simulink model "Model_V5"  (R2024b)
settings: Solver=VariableStepAuto  StartTime=0.0  StopTime=3600*12  RelTol=1e-3
undefined symbols (not defined in the file): PropsSI
libraries: fl_lib x569, SimscapeFluids_lib x61, nesl_utility x27
(part 4 of 7)

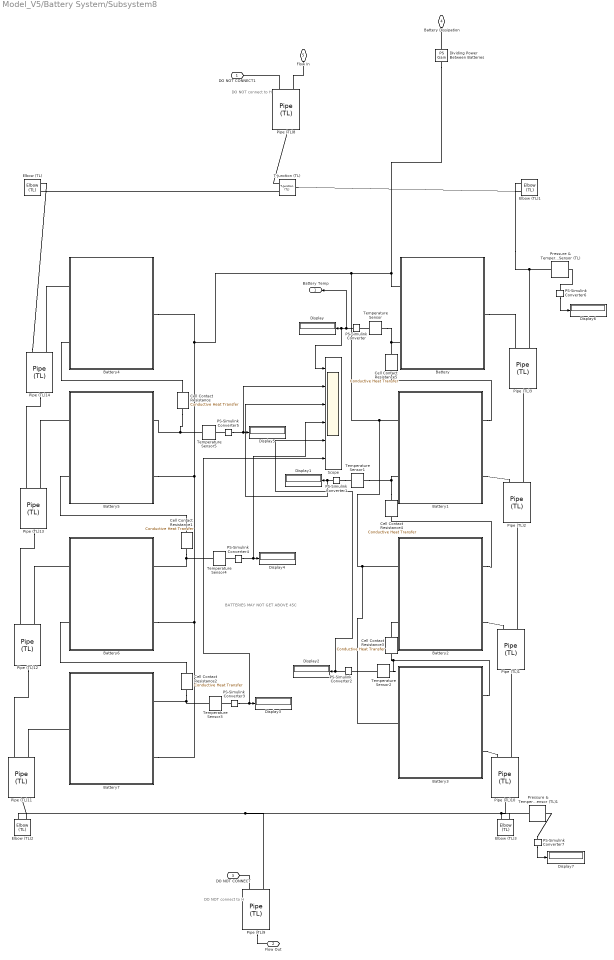
== system Model_V5/Battery System/Subsystem8 ==
  note: BATTERIES MAY NOT GET ABOVE 45C
  note: DO NOT connect to H
  note: DO NOT connect to H
  Battery : Subsystem
      settings: PortSchema="{\"entries\":[{\"content\":{\"sides\":[{\"content\":{},\"type\":\"ConnectorPlacement.EquallySpacedRectSide\",\"uuid\":\"c3611117-ee8e-4b0c-a918-53f59eb75c39\"},{\"content\":{\"side\":\"RIGHT\"},\"type\":\"ConnectorPlacement.EquallySpacedRectSide\",\"uuid\":\"d30ab4df-cb16-40c1-971c-28ba623de8c6\"},{\"content\":{\"connectorIds\":[\"LConn1\",\"LConn2\"],\"side\":\"TOP\"},\"type\":\"ConnectorPlacement.EquallySpacedRectSide\",\"uuid\":\"583a14bc-e521-4cb2-80b3-70b113bba0cc\"},{\"content\":{\"connectorIds\":[\"RConn1\"],\"side\":\"BOTTOM\"},\"type\":\"ConnectorPlacement.EquallySpacedRectSide\",\"uuid\":\"e76e2aad-c8ca-4e56-91e9-6eb1fa374ff6\"}]},\"type\":\"ConnectorPlacement.EquallySpacedConnector\",\"uuid\":\"b27f219d-6435-4727-95fa-791c0451b06d\"}],\"packageUris\":[\"http://schema.mathworks.com/mf0/Connector/R2020b\"],\"version\":\"1.0\"}"
  Battery1 : Subsystem
      settings: PortSchema="{\"entries\":[{\"content\":{\"sides\":[{\"content\":{},\"type\":\"ConnectorPlacement.EquallySpacedRectSide\",\"uuid\":\"c3611117-ee8e-4b0c-a918-53f59eb75c39\"},{\"content\":{\"side\":\"RIGHT\"},\"type\":\"ConnectorPlacement.EquallySpacedRectSide\",\"uuid\":\"d30ab4df-cb16-40c1-971c-28ba623de8c6\"},{\"content\":{\"connectorIds\":[\"LConn1\",\"LConn2\"],\"side\":\"TOP\"},\"type\":\"ConnectorPlacement.EquallySpacedRectSide\",\"uuid\":\"583a14bc-e521-4cb2-80b3-70b113bba0cc\"},{\"content\":{\"connectorIds\":[\"RConn1\",\"RConn2\"],\"side\":\"BOTTOM\"},\"type\":\"ConnectorPlacement.EquallySpacedRectSide\",\"uuid\":\"e76e2aad-c8ca-4e56-91e9-6eb1fa374ff6\"}]},\"type\":\"ConnectorPlacement.EquallySpacedConnector\",\"uuid\":\"b27f219d-6435-4727-95fa-791c0451b06d\"}],\"packageUris\":[\"http://schema.mathworks.com/mf0/Connector/R2020b\"],\"version\":\"1.0\"}"
  Battery2 : Subsystem
      settings: PortSchema="{\"entries\":[{\"content\":{\"sides\":[{\"content\":{},\"type\":\"ConnectorPlacement.EquallySpacedRectSide\",\"uuid\":\"c3611117-ee8e-4b0c-a918-53f59eb75c39\"},{\"content\":{\"side\":\"RIGHT\"},\"type\":\"ConnectorPlacement.EquallySpacedRectSide\",\"uuid\":\"d30ab4df-cb16-40c1-971c-28ba623de8c6\"},{\"content\":{\"connectorIds\":[\"LConn1\",\"LConn2\"],\"side\":\"TOP\"},\"type\":\"ConnectorPlacement.EquallySpacedRectSide\",\"uuid\":\"583a14bc-e521-4cb2-80b3-70b113bba0cc\"},{\"content\":{\"connectorIds\":[\"RConn1\",\"RConn2\"],\"side\":\"BOTTOM\"},\"type\":\"ConnectorPlacement.EquallySpacedRectSide\",\"uuid\":\"e76e2aad-c8ca-4e56-91e9-6eb1fa374ff6\"}]},\"type\":\"ConnectorPlacement.EquallySpacedConnector\",\"uuid\":\"b27f219d-6435-4727-95fa-791c0451b06d\"}],\"packageUris\":[\"http://schema.mathworks.com/mf0/Connector/R2020b\"],\"version\":\"1.0\"}"
  Battery3 : Subsystem
      settings: PortSchema="{\"entries\":[{\"content\":{\"sides\":[{\"content\":{},\"type\":\"ConnectorPlacement.EquallySpacedRectSide\",\"uuid\":\"c3611117-ee8e-4b0c-a918-53f59eb75c39\"},{\"content\":{\"side\":\"RIGHT\"},\"type\":\"ConnectorPlacement.EquallySpacedRectSide\",\"uuid\":\"d30ab4df-cb16-40c1-971c-28ba623de8c6\"},{\"content\":{\"connectorIds\":[\"LConn1\"],\"side\":\"TOP\"},\"type\":\"ConnectorPlacement.EquallySpacedRectSide\",\"uuid\":\"583a14bc-e521-4cb2-80b3-70b113bba0cc\"},{\"content\":{\"connectorIds\":[\"RConn1\",\"RConn2\"],\"side\":\"BOTTOM\"},\"type\":\"ConnectorPlacement.EquallySpacedRectSide\",\"uuid\":\"e76e2aad-c8ca-4e56-91e9-6eb1fa374ff6\"}]},\"type\":\"ConnectorPlacement.EquallySpacedConnector\",\"uuid\":\"b27f219d-6435-4727-95fa-791c0451b06d\"}],\"packageUris\":[\"http://schema.mathworks.com/mf0/Connector/R2020b\"],\"version\":\"1.0\"}"
  Battery4 : Subsystem
      settings: PortSchema="{\"entries\":[{\"content\":{\"sides\":[{\"content\":{},\"type\":\"ConnectorPlacement.EquallySpacedRectSide\",\"uuid\":\"c3611117-ee8e-4b0c-a918-53f59eb75c39\"},{\"content\":{\"side\":\"RIGHT\"},\"type\":\"ConnectorPlacement.EquallySpacedRectSide\",\"uuid\":\"d30ab4df-cb16-40c1-971c-28ba623de8c6\"},{\"content\":{\"connectorIds\":[\"LConn1\"],\"side\":\"TOP\"},\"type\":\"ConnectorPlacement.EquallySpacedRectSide\",\"uuid\":\"583a14bc-e521-4cb2-80b3-70b113bba0cc\"},{\"content\":{\"connectorIds\":[\"RConn1\",\"RConn2\"],\"side\":\"BOTTOM\"},\"type\":\"ConnectorPlacement.EquallySpacedRectSide\",\"uuid\":\"e76e2aad-c8ca-4e56-91e9-6eb1fa374ff6\"}]},\"type\":\"ConnectorPlacement.EquallySpacedConnector\",\"uuid\":\"b27f219d-6435-4727-95fa-791c0451b06d\"}],\"packageUris\":[\"http://schema.mathworks.com/mf0/Connector/R2020b\"],\"version\":\"1.0\"}"
  Battery5 : Subsystem
      settings: PortSchema="{\"entries\":[{\"content\":{\"sides\":[{\"content\":{},\"type\":\"ConnectorPlacement.EquallySpacedRectSide\",\"uuid\":\"c3611117-ee8e-4b0c-a918-53f59eb75c39\"},{\"content\":{\"side\":\"RIGHT\"},\"type\":\"ConnectorPlacement.EquallySpacedRectSide\",\"uuid\":\"d30ab4df-cb16-40c1-971c-28ba623de8c6\"},{\"content\":{\"connectorIds\":[\"LConn1\",\"LConn2\"],\"side\":\"TOP\"},\"type\":\"ConnectorPlacement.EquallySpacedRectSide\",\"uuid\":\"583a14bc-e521-4cb2-80b3-70b113bba0cc\"},{\"content\":{\"connectorIds\":[\"RConn1\",\"RConn2\"],\"side\":\"BOTTOM\"},\"type\":\"ConnectorPlacement.EquallySpacedRectSide\",\"uuid\":\"e76e2aad-c8ca-4e56-91e9-6eb1fa374ff6\"}]},\"type\":\"ConnectorPlacement.EquallySpacedConnector\",\"uuid\":\"b27f219d-6435-4727-95fa-791c0451b06d\"}],\"packageUris\":[\"http://schema.mathworks.com/mf0/Connector/R2020b\"],\"version\":\"1.0\"}"
  Battery6 : Subsystem
      settings: PortSchema="{\"entries\":[{\"content\":{\"sides\":[{\"content\":{},\"type\":\"ConnectorPlacement.EquallySpacedRectSide\",\"uuid\":\"c3611117-ee8e-4b0c-a918-53f59eb75c39\"},{\"content\":{\"side\":\"RIGHT\"},\"type\":\"ConnectorPlacement.EquallySpacedRectSide\",\"uuid\":\"d30ab4df-cb16-40c1-971c-28ba623de8c6\"},{\"content\":{\"connectorIds\":[\"LConn1\",\"LConn2\"],\"side\":\"TOP\"},\"type\":\"ConnectorPlacement.EquallySpacedRectSide\",\"uuid\":\"583a14bc-e521-4cb2-80b3-70b113bba0cc\"},{\"content\":{\"connectorIds\":[\"RConn1\",\"RConn2\"],\"side\":\"BOTTOM\"},\"type\":\"ConnectorPlacement.EquallySpacedRectSide\",\"uuid\":\"e76e2aad-c8ca-4e56-91e9-6eb1fa374ff6\"}]},\"type\":\"ConnectorPlacement.EquallySpacedConnector\",\"uuid\":\"b27f219d-6435-4727-95fa-791c0451b06d\"}],\"packageUris\":[\"http://schema.mathworks.com/mf0/Connector/R2020b\"],\"version\":\"1.0\"}"
  Battery7 : Subsystem
      settings: PortSchema="{\"entries\":[{\"content\":{\"sides\":[{\"content\":{},\"type\":\"ConnectorPlacement.EquallySpacedRectSide\",\"uuid\":\"c3611117-ee8e-4b0c-a918-53f59eb75c39\"},{\"content\":{\"side\":\"RIGHT\"},\"type\":\"ConnectorPlacement.EquallySpacedRectSide\",\"uuid\":\"d30ab4df-cb16-40c1-971c-28ba623de8c6\"},{\"content\":{\"connectorIds\":[\"LConn1\",\"LConn2\"],\"side\":\"TOP\"},\"type\":\"ConnectorPlacement.EquallySpacedRectSide\",\"uuid\":\"583a14bc-e521-4cb2-80b3-70b113bba0cc\"},{\"content\":{\"connectorIds\":[\"RConn1\"],\"side\":\"BOTTOM\"},\"type\":\"ConnectorPlacement.EquallySpacedRectSide\",\"uuid\":\"e76e2aad-c8ca-4e56-91e9-6eb1fa374ff6\"}]},\"type\":\"ConnectorPlacement.EquallySpacedConnector\",\"uuid\":\"b27f219d-6435-4727-95fa-791c0451b06d\"}],\"packageUris\":[\"http://schema.mathworks.com/mf0/Connector/R2020b\"],\"version\":\"1.0\"}"
  Cell Contact Resistance{,1..5} (6 alike) : fl_lib/Thermal/Thermal Elements/Conductive Heat Transfer  thermal_type=foundation.enum.ConstantVariableTabulated.Constant  wall_geometry=foundation.enum.ConductionWallGeometry.Planar  area=12*12 mm^2  thickness=0.003 in  d_in=0.05 m  d_out=0.1 m  L=1 m  th_cond_min=10 W/(K*m)  th_cond=1.38 W/(K*m)  th_cond_TLU=[413, 401, 392, 383, 371, 357, 342] W/(K*m)  temp_TLU=[200, 273, 400, 600, 800, 1000, 1200] K  T_specify=off  T_priority=None  T=0 K  T_nominal_specify=off  T_nominal_value=1  T_nominal_unit=K  Q_specify=off  Q_priority=None  Q=0 W  Q_nominal_specify=off  Q_nominal_value=1  Q_nominal_unit=W
  Display{,1..7} (8 alike) : Display
  Dividing Power Between Batteries : fl_lib/Physical Signals/Functions/PS Gain  gain=1/8
  Elbow (TL){,1..3} (4 alike) : SimscapeFluids_lib/Thermal Liquid/Pipes & Fittings/Elbow (TL)  elbow_type=fluids.thermal_liquid.pipes_fittings.enum.ElbowType.Smooth  diameter_elbow=1.5 in  angle_elbow=90 deg  Re_c=150
      settings: InternalSimscapePortConfiguration="{\"Bottom\":[],\"Left\":[{\"id\":\"A\",\"label\":\"A\",\"type\":\"foundation.thermal_liquid.thermal_liquid\"}],\"Right\":[],\"Top\":[{\"id\":\"B\",\"label\":\"B\",\"type\":\"foundation.thermal_liquid.thermal_liquid\"}]}"
  PS-Simulink Converter{,1..7} (8 alike) : nesl_utility/PS-Simulink Converter  PhysicalDomain=network_engine_domain  SubClassName=ps_output  LeftPortType=input  RightPortType=output  PseudoPeriodic=off  Frequencies=[]  VectorFormat=inherit  Unit=degC  AffineConversion=on
  Pipe (TL)1 : fl_lib/Thermal Liquid/Elements/Pipe (TL)  length=5*301.576 mm  area=5*(99.7+500)*(500+11.6) mm^2  Dh=(10*(99.7+500)*(500+11.6))/((5*(11.6+500))+(99.7+500)) mm  length_add=1 m  roughness=15e-6 m  Re_lam=2000  Re_tur=4000  shape_factor=64  Nu_lam=3.66  dynamic_compressibility=true  inertia=false  p0=0.101325 MPa  T0=293.15 K  mdot0=0 kg/s
  Pipe (TL){10..14} (5 alike) : fl_lib/Thermal Liquid/Elements/Pipe (TL)  length=301.576*5 mm  area=5*(99.7+500)*(500+11.6) mm^2  Dh=(10*(99.7+500)*(500+11.6))/((5*(11.6+500))+(99.7+500)) mm  length_add=1 m  roughness=15e-6 m  Re_lam=2000  Re_tur=4000  shape_factor=64  Nu_lam=3.66  dynamic_compressibility=true  inertia=false  p0=0.101325 MPa  T0=293.15 K  mdot0=0 kg/s
  Pipe (TL)2 : fl_lib/Thermal Liquid/Elements/Pipe (TL)  length=5*301.576 mm  area=5*(99.7+500)*(500+11.6) mm^2  Dh=(10*(99.7+500)*(500+11.6))/((5*(11.6+500))+(99.7+500)) mm  length_add=1 m  roughness=15e-6 m  Re_lam=2000  Re_tur=4000  shape_factor=64  Nu_lam=3.66  dynamic_compressibility=true  inertia=false  p0=0.101325 MPa  T0=293.15 K  mdot0=0 kg/s
  Pipe (TL)3 : fl_lib/Thermal Liquid/Elements/Pipe (TL)  length=5*301.576 mm  area=5*(99.7+500)*(500+11.6) mm^2  Dh=(10*(99.7+500)*(500+11.6))/((5*(11.6+500))+(99.7+500)) mm  length_add=1 m  roughness=15e-6 m  Re_lam=2000  Re_tur=4000  shape_factor=64  Nu_lam=3.66  dynamic_compressibility=true  inertia=false  p0=0.101325 MPa  T0=293.15 K  mdot0=0 kg/s
  Pipe (TL)8 : fl_lib/Thermal Liquid/Elements/Pipe (TL)  length=5 m  area=0.01 m^2  Dh=0.1128 m  length_add=1 m  roughness=15e-6 m  Re_lam=2000  Re_tur=4000  shape_factor=64  Nu_lam=3.66  dynamic_compressibility=true  inertia=false  p0=0.101325 MPa  T0=293.15 K  mdot0=0 kg/s
  Pipe (TL)9 : fl_lib/Thermal Liquid/Elements/Pipe (TL)  length=5 m  area=0.01 m^2  Dh=0.1128 m  length_add=1 m  roughness=15e-6 m  Re_lam=2000  Re_tur=4000  shape_factor=64  Nu_lam=3.66  dynamic_compressibility=true  inertia=false  p0=0.101325 MPa  T0=293.15 K  mdot0=0 kg/s
  Pressure & Temperature Sensor (TL) : fl_lib/Thermal Liquid/Sensors/Pressure & Temperature Sensor (TL)  reference=foundation.enum.MeasurementReference.absolute  pressure=false  pressure_spec=foundation.enum.PressureMeasementSpec.Absolute  temperature=true
      settings: InternalSimscapePortConfiguration="{\"Bottom\":[{\"id\":\"T\",\"label\":\"T\",\"type\":\"output\"}],\"Left\":[{\"id\":\"A\",\"label\":\"A\",\"type\":\"foundation.thermal_liquid.thermal_liquid\"}],\"Right\":[],\"Top\":[]}"
  Pressure & Temperature Sensor (TL)1 : fl_lib/Thermal Liquid/Sensors/Pressure & Temperature Sensor (TL)  reference=foundation.enum.MeasurementReference.absolute  pressure=false  pressure_spec=foundation.enum.PressureMeasementSpec.Absolute  temperature=true
      settings: InternalSimscapePortConfiguration="{\"Bottom\":[{\"id\":\"T\",\"label\":\"T\",\"type\":\"output\"}],\"Left\":[{\"id\":\"A\",\"label\":\"A\",\"type\":\"foundation.thermal_liquid.thermal_liquid\"}],\"Right\":[],\"Top\":[]}"
  Scope : Scope  NumInputPorts=6
  T-Junction (TL) : SimscapeFluids_lib/Thermal Liquid/Pipes & Fittings/T-Junction (TL)  area_main=0.0011 m^2  area_branch=0.0011 m^2  junction_spec=fluids.thermal_liquid.pipes_fittings.enum.TLossCoefficientModel.Crane  k_main_converge=1.12  k_main_diverge=1.12  k_branch_converge=1.12  k_branch_diverge=1.12  loss_coeff_A=1  loss_coeff_B=1  loss_coeff_C=1  radius=0.001 m  Re_c=150  Re_0=10  tau=0.0001 s  saturation_ratio=0.2  smoothing_factor=0.01  inertia=false
      settings: InternalSimscapePortConfiguration="{\"Bottom\":[{\"id\":\"C\",\"label\":\"C\",\"type\":\"foundation.thermal_liquid.thermal_liquid\"}],\"Left\":[{\"id\":\"A\",\"label\":\"A\",\"type\":\"foundation.thermal_liquid.thermal_liquid\"}],\"Right\":[{\"id\":\"B\",\"label\":\"B\",\"type\":\"foundation.thermal_liquid.thermal_liquid\"}],\"Top\":[]}"
  Temperature Sensor{,1..5} (6 alike) : fl_lib/Thermal/Thermal Sensors/Temperature Sensor  temperature_measure=foundation.enum.MeasurementReference.absolute
      settings: InternalSimscapePortConfiguration="{\"Bottom\":[],\"Left\":[{\"id\":\"A\",\"label\":\"A\",\"type\":\"foundation.thermal.thermal\"}],\"Right\":[{\"id\":\"T\",\"label\":\"T\",\"type\":\"output\"}],\"Top\":[]}"
  DO NOT CONNECT1 : PMIOPort  Side=Left
  Flow Out : PMIOPort  Port=2  Side=Left
  DO NOT CONNECT : PMIOPort  Port=3  Side=Left
  Battery Dissipation : PMIOPort  Port=4  Side=Left
  Flow In : PMIOPort  Port=5  Side=Right
  Battery Temp : Outport
  wires:
  PS-Simulink Converter/1 -> Battery Temp/1, Scope/1, Display/1
  PS-Simulink Converter1/1 -> Scope/3, Display1/1
  PS-Simulink Converter2/1 -> Scope/5, Display2/1
  PS-Simulink Converter3/1 -> Scope/6, Display3/1
  PS-Simulink Converter4/1 -> Scope/4, Display4/1
  PS-Simulink Converter5/1 -> Scope/2, Display5/1
  PS-Simulink Converter6/1 -> Display6/1
  PS-Simulink Converter7/1 -> Display7/1
  connections:
  Cell Contact Resistance/RConn1 -- Battery5/LConn1 -- Temperature Sensor5/LConn1
  Pipe (TL)11/LConn2 -- Battery7/RConn1
  Battery3/RConn2 -- Pipe (TL)10/LConn2
  Battery5/RConn2 -- Cell Contact Resistance1/LConn1
  Cell Contact Resistance3/LConn1 -- Battery2/LConn2
  Battery1/RConn1 -- Cell Contact Resistance5/RConn1
  Pipe (TL)10/LConn1 -- Pipe (TL)1/RConn1
  Battery/RConn1 -- Pipe (TL)3/LConn2
  Battery2/RConn2 -- Pipe (TL)1/LConn2
  Cell Contact Resistance4/LConn1 -- Battery1/LConn2 -- Temperature Sensor1/LConn1
  Pipe (TL)1/LConn1 -- Pipe (TL)2/RConn1
  Battery6/RConn1 -- Pipe (TL)12/LConn2
  Cell Contact Resistance2/RConn1 -- Temperature Sensor3/LConn1 -- Battery7/LConn1
  Cell Contact Resistance1/RConn1 -- Battery6/LConn1 -- Temperature Sensor4/LConn1
  Pipe (TL)14/RConn1 -- Pipe (TL)13/LConn1
  Pipe (TL)12/RConn1 -- Pipe (TL)11/LConn1
  Battery4/RConn1 -- Pipe (TL)14/LConn2
  Pipe (TL)8/LConn1 -- Flow In/RConn1
  Battery4/RConn2 -- Cell Contact Resistance/LConn1
  Battery5/RConn1 -- Pipe (TL)13/LConn2
  Pipe (TL)9/LConn2 -- DO NOT CONNECT/RConn1
  Battery2/RConn1 -- Cell Contact Resistance4/RConn1
  Pipe (TL)13/RConn1 -- Pipe (TL)12/LConn1
  Battery1/RConn2 -- Pipe (TL)2/LConn2
  Cell Contact Resistance3/RConn1 -- Battery3/RConn1 -- Temperature Sensor2/LConn1
  Pipe (TL)8/LConn2 -- DO NOT CONNECT1/RConn1
  Pipe (TL)2/LConn1 -- Pipe (TL)3/RConn1
  Battery6/RConn2 -- Cell Contact Resistance2/LConn1
  Battery/LConn2 -- Temperature Sensor/LConn1 -- Cell Contact Resistance5/LConn1
  Pipe (TL)9/RConn1 -- Flow Out/RConn1
  Temperature Sensor/RConn1 -- PS-Simulink Converter/LConn1
  PS-Simulink Converter1/LConn1 -- Temperature Sensor1/RConn1
  PS-Simulink Converter2/LConn1 -- Temperature Sensor2/RConn1
  PS-Simulink Converter3/LConn1 -- Temperature Sensor3/RConn1
  PS-Simulink Converter4/LConn1 -- Temperature Sensor4/RConn1
  PS-Simulink Converter5/LConn1 -- Temperature Sensor5/RConn1
  Dividing Power Between Batteries/LConn1 -- Battery Dissipation/RConn1
  Dividing Power Between Batteries/RConn1 -- Battery3/LConn1 -- Battery2/LConn1 -- Battery1/LConn1 -- Battery7/LConn2 -- Battery6/LConn2 -- Battery5/LConn2 -- Battery4/LConn1 -- Battery/LConn1
  PS-Simulink Converter6/LConn1 -- Pressure & Temperature Sensor (TL)/RConn1
  Pressure & Temperature Sensor (TL)1/RConn1 -- PS-Simulink Converter7/LConn1
  T-Junction (TL)/RConn2 -- Pipe (TL)8/RConn1
  Pressure & Temperature Sensor (TL)/LConn1 -- Pipe (TL)3/LConn1 -- Elbow (TL)1/LConn2
  Elbow (TL)/LConn1 -- T-Junction (TL)/RConn1
  Elbow (TL)1/LConn1 -- T-Junction (TL)/LConn1
  Elbow (TL)/LConn2 -- Pipe (TL)14/LConn1
  Elbow (TL)2/LConn2 -- Elbow (TL)3/LConn2 -- Pipe (TL)9/LConn1
  Elbow (TL)2/LConn1 -- Pipe (TL)11/RConn1
  Elbow (TL)3/LConn1 -- Pipe (TL)10/RConn1 -- Pressure & Temperature Sensor (TL)1/LConn1

== system Model_V5/Engine-Gearbox System/Efficiency Subsystem ==
  (1-Efficiency) Gain : fl_lib/Physical Signals/Functions/PS Product
  PS Constant : fl_lib/Physical Signals/Sources/PS Constant  constant=1
  PS Subtract : fl_lib/Physical Signals/Functions/PS Subtract
  Efficiency : PMIOPort  Side=Left
  Power In : PMIOPort  Port=2  Side=Left
  Heat Dissipation : PMIOPort  Port=3  Side=Right
  connections:
  Power In/RConn1 -- (1-Efficiency) Gain/LConn1
  PS Constant/RConn1 -- PS Subtract/LConn1
  Efficiency/RConn1 -- PS Subtract/LConn2
  PS Subtract/RConn1 -- (1-Efficiency) Gain/LConn2
  Heat Dissipation/RConn1 -- (1-Efficiency) Gain/RConn1

== system Model_V5/HVAC/Ext. Forced h ==
  note: α
  70 degF (degC) : fl_lib/Physical Signals/Sources/PS Constant  constant=(70-32)/1.8+273 K
  Air Properties : Subsystem
  Delay : fl_lib/Physical Signals/Delays/PS Constant Delay  InputHistory=0.5 W/m^2/K  DelayTime=1.0 s
      settings: InternalSimscapePortConfiguration="{\"Bottom\":[],\"Left\":[{\"id\":\"U\",\"label\":\"U\",\"type\":\"input\"}],\"Right\":[{\"id\":\"Y\",\"label\":\"Y\",\"type\":\"output\"}],\"Top\":[]}"
  Nu k : fl_lib/Physical Signals/Functions/PS Product
  Nu k/L : fl_lib/Physical Signals/Functions/PS Gain  gain=1/10 1/m
  Nusselt Number : fl_lib/Physical Signals/Lookup Tables/PS Lookup Table (2D)  x1=10^5:10^5:10^8  x2=[0.7:0.1:20]  f=(0.037*(([10^5:10^5:10^8]').^(4/5) - 5e5.^(4/5)) - 0.664*5e5.^(1/2)).*([0.7:0.1:20]).^(1/3)  interp_method=simscape.enum.interpolation.smooth  extrap_method=simscape.enum.extrapolation.nearest
  Reynolds Number : Subsystem
  Tf : fl_lib/Physical Signals/Functions/PS Gain  gain=0.5
  Ts + Tinf : fl_lib/Physical Signals/Functions/PS Add
  Tair : PMIOPort  Side=Left
  h : PMIOPort  Port=2  Side=Right
  v : PMIOPort  Port=3  Side=Left
  connections:
  Nusselt Number/LConn1 -- Reynolds Number/RConn1
  Nusselt Number/LConn2 -- Air Properties/RConn3
  Delay/LConn1 -- Nu k/L/RConn1
  Nu k/LConn1 -- Nusselt Number/RConn1
  Reynolds Number/LConn2 -- Air Properties/RConn1
  Nu k/L/LConn1 -- Nu k/RConn1
  Delay/RConn1 -- h/RConn1
  Nu k/LConn2 -- Air Properties/RConn4
  Air Properties/RConn2 -- Reynolds Number/LConn3
  Tair/RConn1 -- Ts + Tinf/LConn2
  Tf/LConn1 -- Ts + Tinf/RConn1
  Tf/RConn1 -- Air Properties/LConn1
  70 degF (degC)/RConn1 -- Ts + Tinf/LConn1
  v/RConn1 -- Reynolds Number/LConn1

== system Model_V5/HVAC/Ext. Natural h ==
  note: α
  Air Properties : Subsystem
  Delay : fl_lib/Physical Signals/Delays/PS Constant Delay  InputHistory=0.5 W/m^2/K  DelayTime=1.0 s
      settings: InternalSimscapePortConfiguration="{\"Bottom\":[],\"Left\":[{\"id\":\"U\",\"label\":\"U\",\"type\":\"input\"}],\"Right\":[{\"id\":\"Y\",\"label\":\"Y\",\"type\":\"output\"}],\"Top\":[]}"
  Nu k : fl_lib/Physical Signals/Functions/PS Product
  Nu k/L : fl_lib/Physical Signals/Functions/PS Gain  gain=1/14 1/ft
  Nusselt Number : fl_lib/Physical Signals/Lookup Tables/PS Lookup Table (2D)  x1=[10^4:10^9:10^13]  x2=[0.7:0.1:20]  f=(0.825 + (0.387*([10^4:10^9:10^13]').^(1/6))./(1 + (0.492./([0.7:0.1:20]).^(9/16)).^(8/27))).^2  interp_method=simscape.enum.interpolation.smooth  extrap_method=simscape.enum.extrapolation.nearest
  Rayleigh Number : Subsystem
      settings: PortSchema="{\"entries\":[{\"content\":{\"sides\":[{\"content\":{\"connectorIds\":[\"LConn1\",\"LConn2\",\"LConn3\"]},\"type\":\"ConnectorPlacement.EquallySpacedRectSide\",\"uuid\":\"ae5f1cb6-4634-4289-8b16-d6c06926f572\"},{\"content\":{\"connectorIds\":[\"RConn1\"],\"side\":\"RIGHT\"},\"type\":\"ConnectorPlacement.EquallySpacedRectSide\",\"uuid\":\"887b4ef1-1011-48e9-a0f3-0c26976b5a26\"},{\"content\":{\"connectorIds\":[\"LConn4\",\"LConn5\"],\"side\":\"TOP\"},\"type\":\"ConnectorPlacement.EquallySpacedRectSide\",\"uuid\":\"f0a29ad1-7357-4b54-ad18-1d423d3cc700\"}]},\"type\":\"ConnectorPlacement.EquallySpacedConnector\",\"uuid\":\"e8da6873-c4bf-48bb-b6e2-8ce26624a058\"}],\"packageUris\":[\"http://schema.mathworks.com/mf0/Connector/R2020b\"],\"version\":\"1.0\"}"
  Tf : fl_lib/Physical Signals/Functions/PS Gain  gain=0.5
  Ts + Tair : fl_lib/Physical Signals/Functions/PS Add
  Ts : PMIOPort  Side=Left
  h : PMIOPort  Port=2  Side=Right
  Tair : PMIOPort  Port=3  Side=Left
  connections:
  Ts + Tair/LConn1 -- Rayleigh Number/LConn4 -- Ts/RConn1
  Rayleigh Number/LConn5 -- Ts + Tair/LConn2 -- Tair/RConn1
  Tf/LConn1 -- Ts + Tair/RConn1
  Tf/RConn1 -- Air Properties/LConn1
  Rayleigh Number/LConn1 -- Air Properties/RConn1
  Rayleigh Number/LConn2 -- Air Properties/RConn2
  Air Properties/RConn3 -- Rayleigh Number/LConn3
  Nusselt Number/LConn1 -- Rayleigh Number/RConn1
  Nusselt Number/LConn2 -- Air Properties/RConn4
  Nu k/LConn1 -- Nusselt Number/RConn1
  Nu k/LConn2 -- Air Properties/RConn5
  Nu k/L/LConn1 -- Nu k/RConn1
  Delay/LConn1 -- Nu k/L/RConn1
  Delay/RConn1 -- h/RConn1

== system Model_V5/HVAC/Gs ==
  note: Solar Zenith Angle
  note: Solar Load
  90 deg : fl_lib/Physical Signals/Sources/PS Constant  constant=90 deg
  Convert to deg : fl_lib/Physical Signals/Functions/PS Gain  gain=90 deg
  Direct Solar : fl_lib/Physical Signals/Functions/PS Product
  Front Window Top-down Area : fl_lib/Physical Signals/Functions/PS Gain  gain=55*40*0.5 in^2
  PS Add1 : fl_lib/Physical Signals/Functions/PS Add
  PS Saturation : fl_lib/Physical Signals/Nonlinear Operators/PS Saturation  upper_limit=1  lower_limit=0.7
  PS Saturation2 : fl_lib/Physical Signals/Nonlinear Operators/PS Saturation  upper_limit=1  lower_limit=0.7
  PS Sine Wave : fl_lib/Physical Signals/Sources/PS Sine Wave  amplitude=1  bias=0  frequency_spec=foundation.enum.frequencySpec.angular  frequency_SI=1 Hz  frequency_angular=pi/24 rad/hr  phase=pi/4 rad
      settings: InternalSimscapePortConfiguration="{\"Bottom\":[],\"Left\":[],\"Right\":[{\"id\":\"O\",\"label\":\"\",\"type\":\"output\"}],\"Top\":[]}"
  PS Sine Wave2 : fl_lib/Physical Signals/Sources/PS Sine Wave  amplitude=1  bias=0  frequency_spec=foundation.enum.frequencySpec.angular  frequency_SI=1 Hz  frequency_angular=pi/24 rad/hr  phase=pi/4 rad
      settings: InternalSimscapePortConfiguration="{\"Bottom\":[],\"Left\":[],\"Right\":[{\"id\":\"O\",\"label\":\"\",\"type\":\"output\"}],\"Top\":[]}"
  PS Step : fl_lib/Physical Signals/Sources/PS Step  step_time=3600*6 s  initial_value=0  final_value=1
  PS Subtract1 : fl_lib/Physical Signals/Functions/PS Subtract
  PS Switch : fl_lib/Physical Signals/Nonlinear Operators/PS Switch  Threshold=0.5
      settings: InternalSimscapePortConfiguration="{\"Bottom\":[],\"Left\":[{\"id\":\"I1\",\"label\":\"\",\"type\":\"input\"},{\"id\":\"I2\",\"label\":\"\",\"type\":\"input\"},{\"id\":\"I3\",\"label\":\"\",\"type\":\"input\"}],\"Right\":[{\"id\":\"O\",\"label\":\"\",\"type\":\"output\"}],\"Top\":[]}"
  Solar Irradiance : fl_lib/Physical Signals/Functions/PS Gain  gain=1414 W/m^2
  Total Window Areas : fl_lib/Physical Signals/Functions/PS Gain  gain=55*40+40*40+40*40 in^2
  Window Angle : fl_lib/Physical Signals/Sources/PS Constant  constant=120 deg
  cos(w-s) : fl_lib/Physical Signals/Functions/PS Math Function  fcn_choice=foundation.enum.math_function.cos  v=1
  ρ : fl_lib/Physical Signals/Functions/PS Gain  gain=0.20
  Gs : PMIOPort  Side=Right
  connections:
  PS Saturation2/RConn1 -- Convert to deg/LConn1
  ρ/LConn1 -- Total Window Areas/RConn1
  Front Window Top-down Area/RConn1 -- Direct Solar/LConn2
  PS Sine Wave2/RConn1 -- PS Saturation2/LConn1
  PS Sine Wave/RConn1 -- PS Saturation/LConn1
  Solar Irradiance/LConn1 -- PS Saturation/RConn1
  PS Subtract1/RConn1 -- PS Switch/LConn3
  PS Switch/RConn1 -- cos(w-s)/LConn1
  PS Add1/LConn1 -- ρ/RConn1
  PS Add1/LConn2 -- Direct Solar/RConn1
  90 deg/RConn1 -- PS Switch/LConn1
  Window Angle/RConn1 -- PS Subtract1/LConn1
  Convert to deg/RConn1 -- PS Subtract1/LConn2
  PS Add1/RConn1 -- Gs/RConn1
  cos(w-s)/RConn1 -- Front Window Top-down Area/LConn1
  Total Window Areas/LConn1 -- Solar Irradiance/RConn1 -- Direct Solar/LConn1
  PS Step/RConn1 -- PS Switch/LConn2

== system Model_V5/HVAC/HVAC h ==
  note: Use flat plate correlation, where length of plate is double the length of car (L = 221*2 in.)
  note: α
  70 degF (degC) : fl_lib/Physical Signals/Sources/PS Constant  constant=(70-32)/1.8+273 K
  Air Properties : Subsystem
  Delay for Stability : fl_lib/Physical Signals/Delays/PS Constant Delay  InputHistory=0.5 W/m^2/K  DelayTime=1.0 s
      settings: InternalSimscapePortConfiguration="{\"Bottom\":[],\"Left\":[{\"id\":\"U\",\"label\":\"U\",\"type\":\"input\"}],\"Right\":[{\"id\":\"Y\",\"label\":\"Y\",\"type\":\"output\"}],\"Top\":[]}"
  Nu k : fl_lib/Physical Signals/Functions/PS Product
  Nu k/L : fl_lib/Physical Signals/Functions/PS Gain  gain=1/10 1/m
  Nusselt Number : fl_lib/Physical Signals/Lookup Tables/PS Lookup Table (2D)  x1=10^5:10^5:10^8  x2=[0.7:0.1:20]  f=(0.037*(([10^5:10^5:10^8]').^(4/5) - 5e5.^(4/5)) - 0.664*5e5.^(1/2)).*([0.7:0.1:20]).^(1/3)  interp_method=simscape.enum.interpolation.smooth  extrap_method=simscape.enum.extrapolation.nearest
  Reynolds Number : Subsystem
  Tf : fl_lib/Physical Signals/Functions/PS Gain  gain=0.5
  Ts + Tinf : fl_lib/Physical Signals/Functions/PS Add
  Tair : PMIOPort  Side=Left
  h : PMIOPort  Port=2  Side=Right
  connections:
  Reynolds Number/RConn1 -- Nusselt Number/LConn1
  Nusselt Number/LConn2 -- Air Properties/RConn3
  Delay for Stability/LConn1 -- Nu k/L/RConn1
  Nu k/LConn1 -- Nusselt Number/RConn1
  Reynolds Number/LConn1 -- Air Properties/RConn1
  Nu k/L/LConn1 -- Nu k/RConn1
  Delay for Stability/RConn1 -- h/RConn1
  Nu k/LConn2 -- Air Properties/RConn4
  Reynolds Number/LConn2 -- Air Properties/RConn2
  Tair/RConn1 -- Ts + Tinf/LConn2
  Tf/LConn1 -- Ts + Tinf/RConn1
  Tf/RConn1 -- Air Properties/LConn1
  70 degF (degC)/RConn1 -- Ts + Tinf/LConn1

== system Model_V5/HVAC/Text ==
  10 K : fl_lib/Physical Signals/Sources/PS Constant  constant=10 K
  6.8977 K^(1/3) : fl_lib/Physical Signals/Functions/PS Gain  gain=6.8977 K^(1/3)
  Air Temperature : fl_lib/Physical Signals/Functions/PS Gain  gain=40 + 273 K
  PS Saturation1 : fl_lib/Physical Signals/Nonlinear Operators/PS Saturation  upper_limit=1  lower_limit=0.7
  PS Sine Wave1 : fl_lib/Physical Signals/Sources/PS Sine Wave  amplitude=1  bias=0  frequency_spec=foundation.enum.frequencySpec.angular  frequency_SI=1 Hz  frequency_angular=pi/24 rad/hr  phase=pi/4 rad
      settings: InternalSimscapePortConfiguration="{\"Bottom\":[],\"Left\":[],\"Right\":[{\"id\":\"O\",\"label\":\"\",\"type\":\"output\"}],\"Top\":[]}"
  PS Subtract : fl_lib/Physical Signals/Functions/PS Subtract
  T^(2/3) : fl_lib/Physical Signals/Functions/PS Math Function  fcn_choice=foundation.enum.math_function.pow  v=2/3
  Text : PMIOPort  Side=Right
  connections:
  PS Subtract/RConn1 -- T^(2/3)/LConn1
  10 K/RConn1 -- PS Subtract/LConn2
  PS Subtract/LConn1 -- Air Temperature/RConn1
  T^(2/3)/RConn1 -- 6.8977 K^(1/3)/LConn1
  Air Temperature/LConn1 -- PS Saturation1/RConn1
  PS Sine Wave1/RConn1 -- PS Saturation1/LConn1
  6.8977 K^(1/3)/RConn1 -- Text/RConn1

== system Model_V5/HVAC/Window (Front) h ==
  note: α
  Air Properties : Subsystem
  Delay for Stability : fl_lib/Physical Signals/Delays/PS Constant Delay  InputHistory=0.5 W/m^2/K  DelayTime=1.0 s
      settings: InternalSimscapePortConfiguration="{\"Bottom\":[],\"Left\":[{\"id\":\"U\",\"label\":\"U\",\"type\":\"input\"}],\"Right\":[{\"id\":\"Y\",\"label\":\"Y\",\"type\":\"output\"}],\"Top\":[]}"
  Nu k : fl_lib/Physical Signals/Functions/PS Product
  Nu k/L : fl_lib/Physical Signals/Functions/PS Gain  gain=1/14 1/ft
  Nusselt Number : fl_lib/Physical Signals/Lookup Tables/PS Lookup Table (2D)  x1=[10^4:10^9:10^13]  x2=[0.7:0.1:20]  f=(0.825 + (0.387*([10^4:10^9:10^13]').^(1/6))./(1 + (0.492./([0.7:0.1:20]).^(9/16)).^(8/27))).^2  interp_method=simscape.enum.interpolation.smooth  extrap_method=simscape.enum.extrapolation.nearest
  Rayleigh Number : Subsystem
      settings: PortSchema="{\"entries\":[{\"content\":{\"sides\":[{\"content\":{\"connectorIds\":[\"LConn1\",\"LConn2\",\"LConn3\"]},\"type\":\"ConnectorPlacement.EquallySpacedRectSide\",\"uuid\":\"ae5f1cb6-4634-4289-8b16-d6c06926f572\"},{\"content\":{\"connectorIds\":[\"RConn1\"],\"side\":\"RIGHT\"},\"type\":\"ConnectorPlacement.EquallySpacedRectSide\",\"uuid\":\"887b4ef1-1011-48e9-a0f3-0c26976b5a26\"},{\"content\":{\"connectorIds\":[\"LConn4\",\"LConn5\"],\"side\":\"TOP\"},\"type\":\"ConnectorPlacement.EquallySpacedRectSide\",\"uuid\":\"f0a29ad1-7357-4b54-ad18-1d423d3cc700\"}]},\"type\":\"ConnectorPlacement.EquallySpacedConnector\",\"uuid\":\"e8da6873-c4bf-48bb-b6e2-8ce26624a058\"}],\"packageUris\":[\"http://schema.mathworks.com/mf0/Connector/R2020b\"],\"version\":\"1.0\"}"
  Tf : fl_lib/Physical Signals/Functions/PS Gain  gain=0.5
  Ts + Tair : fl_lib/Physical Signals/Functions/PS Add
  Tair : PMIOPort  Side=Left
  Ts : PMIOPort  Port=2  Side=Left
  h : PMIOPort  Port=3  Side=Right
  connections:
  Ts + Tair/LConn1 -- Rayleigh Number/LConn4 -- Ts/RConn1
  Rayleigh Number/LConn5 -- Ts + Tair/LConn2 -- Tair/RConn1
  Tf/LConn1 -- Ts + Tair/RConn1
  Tf/RConn1 -- Air Properties/LConn1
  Rayleigh Number/LConn1 -- Air Properties/RConn1
  Rayleigh Number/LConn2 -- Air Properties/RConn2
  Air Properties/RConn3 -- Rayleigh Number/LConn3
  Nusselt Number/LConn1 -- Rayleigh Number/RConn1
  Nusselt Number/LConn2 -- Air Properties/RConn4
  Nu k/LConn1 -- Nusselt Number/RConn1
  Nu k/LConn2 -- Air Properties/RConn5
  Nu k/L/LConn1 -- Nu k/RConn1
  Delay for Stability/LConn1 -- Nu k/L/RConn1
  Delay for Stability/RConn1 -- h/RConn1

== system Model_V5/HVAC/Window (Side) h ==
  note: α
  Air Properties : Subsystem
  Delay for Stability : fl_lib/Physical Signals/Delays/PS Constant Delay  InputHistory=0.5 W/m^2/K  DelayTime=1.0 s
      settings: InternalSimscapePortConfiguration="{\"Bottom\":[],\"Left\":[{\"id\":\"U\",\"label\":\"U\",\"type\":\"input\"}],\"Right\":[{\"id\":\"Y\",\"label\":\"Y\",\"type\":\"output\"}],\"Top\":[]}"
  Nu k : fl_lib/Physical Signals/Functions/PS Product
  Nu k/L : fl_lib/Physical Signals/Functions/PS Gain  gain=1/14 1/ft
  Nusselt Number : fl_lib/Physical Signals/Lookup Tables/PS Lookup Table (2D)  x1=[10^4:10^9:10^13]  x2=[0.7:0.1:20]  f=(0.825 + (0.387*([10^4:10^9:10^13]').^(1/6))./(1 + (0.492./([0.7:0.1:20]).^(9/16)).^(8/27))).^2  interp_method=simscape.enum.interpolation.smooth  extrap_method=simscape.enum.extrapolation.nearest
  Rayleigh Number : Subsystem
      settings: PortSchema="{\"entries\":[{\"content\":{\"sides\":[{\"content\":{\"connectorIds\":[\"LConn1\",\"LConn2\",\"LConn3\"]},\"type\":\"ConnectorPlacement.EquallySpacedRectSide\",\"uuid\":\"ae5f1cb6-4634-4289-8b16-d6c06926f572\"},{\"content\":{\"connectorIds\":[\"RConn1\"],\"side\":\"RIGHT\"},\"type\":\"ConnectorPlacement.EquallySpacedRectSide\",\"uuid\":\"887b4ef1-1011-48e9-a0f3-0c26976b5a26\"},{\"content\":{\"connectorIds\":[\"LConn4\",\"LConn5\"],\"side\":\"TOP\"},\"type\":\"ConnectorPlacement.EquallySpacedRectSide\",\"uuid\":\"f0a29ad1-7357-4b54-ad18-1d423d3cc700\"}]},\"type\":\"ConnectorPlacement.EquallySpacedConnector\",\"uuid\":\"e8da6873-c4bf-48bb-b6e2-8ce26624a058\"}],\"packageUris\":[\"http://schema.mathworks.com/mf0/Connector/R2020b\"],\"version\":\"1.0\"}"
  Tf : fl_lib/Physical Signals/Functions/PS Gain  gain=0.5
  Ts + Tair : fl_lib/Physical Signals/Functions/PS Add
  Ts : PMIOPort  Side=Left
  h : PMIOPort  Port=2  Side=Right
  Tair : PMIOPort  Port=3  Side=Left
  connections:
  Ts + Tair/LConn1 -- Rayleigh Number/LConn4 -- Ts/RConn1
  Rayleigh Number/LConn5 -- Ts + Tair/LConn2 -- Tair/RConn1
  Tf/LConn1 -- Ts + Tair/RConn1
  Tf/RConn1 -- Air Properties/LConn1
  Rayleigh Number/LConn1 -- Air Properties/RConn1
  Rayleigh Number/LConn2 -- Air Properties/RConn2
  Air Properties/RConn3 -- Rayleigh Number/LConn3
  Nusselt Number/LConn1 -- Rayleigh Number/RConn1
  Nusselt Number/LConn2 -- Air Properties/RConn4
  Nu k/LConn1 -- Nusselt Number/RConn1
  Nu k/LConn2 -- Air Properties/RConn5
  Nu k/L/LConn1 -- Nu k/RConn1
  Delay for Stability/LConn1 -- Nu k/L/RConn1
  Delay for Stability/RConn1 -- h/RConn1

== system Model_V5/Inverter/Efficiency Subsystem ==
  (1-Efficiency) Gain : fl_lib/Physical Signals/Functions/PS Product
  PS Constant : fl_lib/Physical Signals/Sources/PS Constant  constant=1
  PS Subtract : fl_lib/Physical Signals/Functions/PS Subtract
  Efficiency : PMIOPort  Side=Left
  Power In : PMIOPort  Port=2  Side=Left
  Heat Dissipation : PMIOPort  Port=3  Side=Right
  connections:
  Power In/RConn1 -- (1-Efficiency) Gain/LConn1
  PS Constant/RConn1 -- PS Subtract/LConn1
  Efficiency/RConn1 -- PS Subtract/LConn2
  PS Subtract/RConn1 -- (1-Efficiency) Gain/LConn2
  Heat Dissipation/RConn1 -- (1-Efficiency) Gain/RConn1

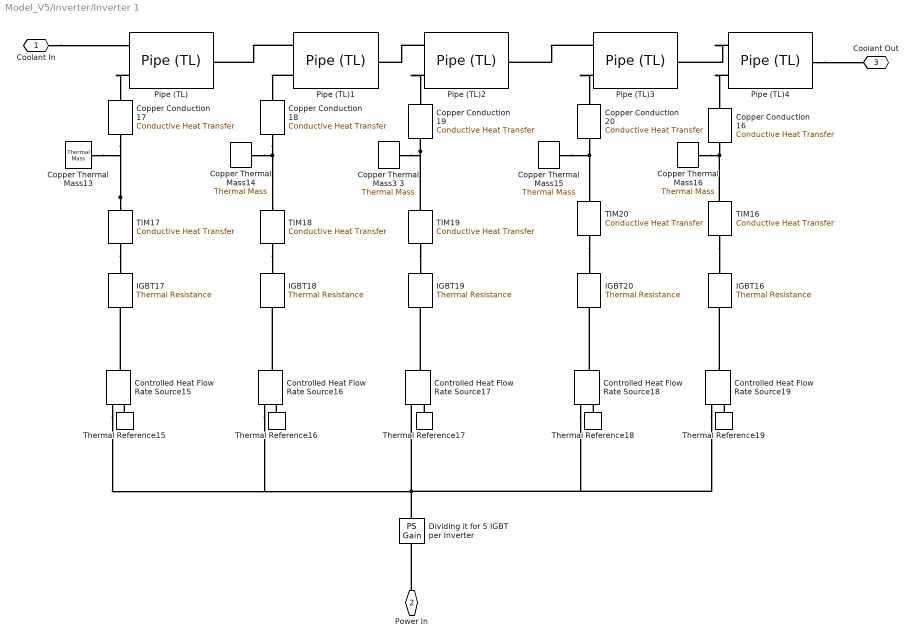
== system Model_V5/Inverter/Inverter 1 ==
  Controlled Heat Flow Rate Source{15..19} (5 alike) : fl_lib/Thermal/Thermal Sources/Controlled Heat Flow Rate Source
  Copper Conduction 16 : fl_lib/Thermal/Thermal Elements/Conductive Heat Transfer  thermal_type=foundation.enum.ConstantVariableTabulated.Constant  wall_geometry=foundation.enum.ConductionWallGeometry.Planar  area=0.03*0.36 m^2  thickness=5 cm  d_in=0.05 m  d_out=0.1 m  L=1 m  th_cond_min=10 W/(K*m)  th_cond=401 W/(K*m)  th_cond_TLU=[413, 401, 392, 383, 371, 357, 342] W/(K*m)  temp_TLU=[200, 273, 400, 600, 800, 1000, 1200] K  T_specify=off  T_priority=None  T=0 K  T_nominal_specify=off  T_nominal_value=1  T_nominal_unit=K  Q_specify=off  Q_priority=None  Q=0 W  Q_nominal_specify=off  Q_nominal_value=1  Q_nominal_unit=W
  Copper Conduction 17 : fl_lib/Thermal/Thermal Elements/Conductive Heat Transfer  thermal_type=foundation.enum.ConstantVariableTabulated.Constant  wall_geometry=foundation.enum.ConductionWallGeometry.Planar  area=0.03*0.36 m^2  thickness=4 cm  d_in=0.05 m  d_out=0.1 m  L=1 m  th_cond_min=10 W/(K*m)  th_cond=401 W/(K*m)  th_cond_TLU=[413, 401, 392, 383, 371, 357, 342] W/(K*m)  temp_TLU=[200, 273, 400, 600, 800, 1000, 1200] K  T_specify=off  T_priority=None  T=0 K  T_nominal_specify=off  T_nominal_value=1  T_nominal_unit=K  Q_specify=off  Q_priority=None  Q=0 W  Q_nominal_specify=off  Q_nominal_value=1  Q_nominal_unit=W
  Copper Conduction 18 : fl_lib/Thermal/Thermal Elements/Conductive Heat Transfer  thermal_type=foundation.enum.ConstantVariableTabulated.Constant  wall_geometry=foundation.enum.ConductionWallGeometry.Planar  area=0.03*0.36 m^2  thickness=2 mm  d_in=0.05 m  d_out=0.1 m  L=1 m  th_cond_min=10 W/(K*m)  th_cond=401 W/(K*m)  th_cond_TLU=[413, 401, 392, 383, 371, 357, 342] W/(K*m)  temp_TLU=[200, 273, 400, 600, 800, 1000, 1200] K  T_specify=off  T_priority=None  T=0 K  T_nominal_specify=off  T_nominal_value=1  T_nominal_unit=K  Q_specify=off  Q_priority=None  Q=0 W  Q_nominal_specify=off  Q_nominal_value=1  Q_nominal_unit=W
  Copper Conduction 19 : fl_lib/Thermal/Thermal Elements/Conductive Heat Transfer  thermal_type=foundation.enum.ConstantVariableTabulated.Constant  wall_geometry=foundation.enum.ConductionWallGeometry.Planar  area=0.03*0.36 m^2  thickness=2 mm  d_in=0.05 m  d_out=0.1 m  L=1 m  th_cond_min=10 W/(K*m)  th_cond=401 W/(K*m)  th_cond_TLU=[413, 401, 392, 383, 371, 357, 342] W/(K*m)  temp_TLU=[200, 273, 400, 600, 800, 1000, 1200] K  T_specify=off  T_priority=None  T=0 K  T_nominal_specify=off  T_nominal_value=1  T_nominal_unit=K  Q_specify=off  Q_priority=None  Q=0 W  Q_nominal_specify=off  Q_nominal_value=1  Q_nominal_unit=W
  Copper Conduction 20 : fl_lib/Thermal/Thermal Elements/Conductive Heat Transfer  thermal_type=foundation.enum.ConstantVariableTabulated.Constant  wall_geometry=foundation.enum.ConductionWallGeometry.Planar  area=0.03*0.36 m^2  thickness=2 mm  d_in=0.05 m  d_out=0.1 m  L=1 m  th_cond_min=10 W/(K*m)  th_cond=401 W/(K*m)  th_cond_TLU=[413, 401, 392, 383, 371, 357, 342] W/(K*m)  temp_TLU=[200, 273, 400, 600, 800, 1000, 1200] K  T_specify=off  T_priority=None  T=0 K  T_nominal_specify=off  T_nominal_value=1  T_nominal_unit=K  Q_specify=off  Q_priority=None  Q=0 W  Q_nominal_specify=off  Q_nominal_value=1  Q_nominal_unit=W
  Copper Thermal Mass13 : fl_lib/Thermal/Thermal Elements/Thermal Mass  mass_type=foundation.enum.constant_variable.constant  mass=6*10^-4*8000 kg  sp_heat=376.812 J/(K*kg)  mass_min=1e-6 kg  num_ports=foundation.enum.numPorts2.one  m_specify=off  m_priority=High  m=1 kg  m_nominal_specify=off  m_nominal_value=1  m_nominal_unit=kg  T_specify=on  T_priority=High  T=292 K  T_nominal_specify=off  T_nominal_value=1  T_nominal_unit=K  Q_specify=off  Q_priority=None  Q=0 W  Q_nominal_specify=off  Q_nominal_value=1  Q_nominal_unit=W
  Copper Thermal Mass14 : fl_lib/Thermal/Thermal Elements/Thermal Mass  mass_type=foundation.enum.constant_variable.constant  mass=7.5*10^-4*8000 kg  sp_heat=376.812 J/(K*kg)  mass_min=1e-6 kg  num_ports=foundation.enum.numPorts2.one  m_specify=off  m_priority=High  m=1 kg  m_nominal_specify=off  m_nominal_value=1  m_nominal_unit=kg  T_specify=on  T_priority=High  T=292 K  T_nominal_specify=off  T_nominal_value=1  T_nominal_unit=K  Q_specify=off  Q_priority=None  Q=0 W  Q_nominal_specify=off  Q_nominal_value=1  Q_nominal_unit=W
  Copper Thermal Mass15 : fl_lib/Thermal/Thermal Elements/Thermal Mass  mass_type=foundation.enum.constant_variable.constant  mass=7.5*10^-4*8000 kg  sp_heat=376.812 J/(K*kg)  mass_min=1e-6 kg  num_ports=foundation.enum.numPorts2.one  m_specify=off  m_priority=High  m=1 kg  m_nominal_specify=off  m_nominal_value=1  m_nominal_unit=kg  T_specify=on  T_priority=High  T=292 K  T_nominal_specify=off  T_nominal_value=1  T_nominal_unit=K  Q_specify=off  Q_priority=None  Q=0 W  Q_nominal_specify=off  Q_nominal_value=1  Q_nominal_unit=W
  Copper Thermal Mass16 : fl_lib/Thermal/Thermal Elements/Thermal Mass  mass_type=foundation.enum.constant_variable.constant  mass=7.5*10^-4*8000 kg  sp_heat=376.812 J/(K*kg)  mass_min=1e-6 kg  num_ports=foundation.enum.numPorts2.one  m_specify=off  m_priority=High  m=1 kg  m_nominal_specify=off  m_nominal_value=1  m_nominal_unit=kg  T_specify=on  T_priority=High  T=292 K  T_nominal_specify=off  T_nominal_value=1  T_nominal_unit=K  Q_specify=off  Q_priority=None  Q=0 W  Q_nominal_specify=off  Q_nominal_value=1  Q_nominal_unit=W
  Copper Thermal Mass3 3 : fl_lib/Thermal/Thermal Elements/Thermal Mass  mass_type=foundation.enum.constant_variable.constant  mass=7.5*10^-4*8000 kg  sp_heat=376.812 J/(K*kg)  mass_min=1e-6 kg  num_ports=foundation.enum.numPorts2.one  m_specify=off  m_priority=High  m=1 kg  m_nominal_specify=off  m_nominal_value=1  m_nominal_unit=kg  T_specify=on  T_priority=High  T=292 K  T_nominal_specify=off  T_nominal_value=1  T_nominal_unit=K  Q_specify=off  Q_priority=None  Q=0 W  Q_nominal_specify=off  Q_nominal_value=1  Q_nominal_unit=W
  Dividing it for 5 IGBT per Inverter : fl_lib/Physical Signals/Functions/PS Gain  gain=1/5
  IGBT{16..20} (5 alike) : fl_lib/Thermal/Thermal Elements/Thermal Resistance  resistance=1/10 K/W  T_specify=off  T_priority=None  T=0 K  T_nominal_specify=off  T_nominal_value=1  T_nominal_unit=K  Q_specify=off  Q_priority=None  Q=0 W  Q_nominal_specify=off  Q_nominal_value=1  Q_nominal_unit=W
  Pipe (TL){,1..4} (5 alike) : SimscapeFluids_lib/Thermal Liquid/Pipes & Fittings/Pipe (TL)  dynamic_compressibility=false  inertia=false  num_segments=1  pipe_length=5*3 cm  cross_section_geometry=fluids.thermal_liquid.pipes_fittings.enum.CrossSectionGeometry.Rectangular  pipe_diameter=0.1 m  pipe_inner_diameter=0.05 m  pipe_outer_diameter=0.1 m  pipe_width=0.35 m  pipe_height=0.004 m  pipe_major_axis=0.1 m  pipe_minor_axis=0.05 m  pipe_side=0.1 m  pipe_angle=30 deg  area=0.01 m^2  Dh=0.1128 m  elevation_spec=foundation.enum.constant_variable.constant  elevation_gain=0 m  gravity_spec=foundation.enum.constant_variable.constant  g=9.81 m/s^2  pressure_loss_spec=fluids.thermal_liquid.pipes_fittings.enum.PressureLossSpec.Haaland  local_pressure_loss_spec=fluids.thermal_liquid.pipes_fittings.enum.LocalLossSpec.AggregateLength  length_add=1 m  loss_coefficient=0.1  roughness_spec=fluids.thermal_liquid.pipes_fittings.enum.RoughnessSpec.CommercialPipe  roughness=15e-6 m  Re_friction_TLU=[400, 1000, 1500, 3000, 4000, 6000, 10000, 20000, 40000, 60000, 100000, 100000000]  friction_factor_TLU=[.264, .112, .071, .0417, .0387, .0268, .025, .0232, .0226, .022, .0214, .0214]  Re_lam=2000  Re_tur=4000  shape_factor=64  mdot_nominal=[.1, 1] kg/s  p_diff_nominal=[.001, .01] MPa  mdot_threshold=1e-6 kg/s  wall_spec=fluids.thermal_liquid.pipes_fittings.enum.wall_spec.rigid  vol_expansion_spec=fluids.thermal_liquid.pipes_fittings.enum.VolumeExpansionSpec.Area  area_pressure_gain=1e-6 m^2/MPa  static_pressure_TLU=[.1, 1] MPa  area_pressure_gain_TLU=[1e-05, 1.1e-05] m^2  material_behavior_spec=fluids.thermal_liquid.pipes_fittings.enum.PipeMaterialBehavior.Linear  diameter_pressure_gain=1e-6 m/MPa  wall_thickness=0.05 m  elastic_modulus=69 GPa  stress_TLU=[276, 310] MPa  strain_TLU=[.004, .02]  stress_assert_action=simscape.enum.assert.action.none  stress_max=400 MPa  poisson_ratio=0.33  wall_time_constant=0.01 s  thermal_expansion=false  alpha_L_wall=24 um/(deltaK*m)  thermal_expansion_Tref=293.15 K  heat_transfer_spec=fluids.thermal_liquid.pipes_fittings.enum.HeatTransferSpec.Gnielinski  mdot_nominal_heat=[.1, 1] kg/s  T_in_nominal=[293.15, 293.15] K  T_out_nominal=[300, 300] K  p_in_nominal_heat=[.101325, .101325] MPa  T_wall_nominal=[303.15, 303.15] K  a_coeff=0.023  b_Re_power=0.8  c_Pr_power=0.4  Nu_lam=3.66  Re_Colburn_TLU=[100, 150, 1000]  Colburn_factor_TLU=[.019, .013, .002]  Re_Nu_TLU=[100, 150, 1000]  Pr_Nu_TLU=[1, 10]  Nu_TLU=[3.72, 4.21; 3.75, 4.44; 4.21, 7.15]  p0_vec=0.101325 MPa  T0_vec=40+273.15 K  mdot0=0.1 kg/s
  TIM16 : fl_lib/Thermal/Thermal Elements/Conductive Heat Transfer  thermal_type=foundation.enum.ConstantVariableTabulated.Constant  wall_geometry=foundation.enum.ConductionWallGeometry.Planar  area=0.1 m^2  thickness=0.001 in  d_in=0.05 m  d_out=0.1 m  L=1 m  th_cond_min=10 W/(K*m)  th_cond=8.9 W/(K*m)  th_cond_TLU=[413, 401, 392, 383, 371, 357, 342] W/(K*m)  temp_TLU=[200, 273, 400, 600, 800, 1000, 1200] K  T_specify=off  T_priority=None  T=0 K  T_nominal_specify=off  T_nominal_value=1  T_nominal_unit=K  Q_specify=off  Q_priority=None  Q=0 W  Q_nominal_specify=off  Q_nominal_value=1  Q_nominal_unit=W
  TIM17 : fl_lib/Thermal/Thermal Elements/Conductive Heat Transfer  thermal_type=foundation.enum.ConstantVariableTabulated.Constant  wall_geometry=foundation.enum.ConductionWallGeometry.Planar  area=0.01 m^2  thickness=0.001 in  d_in=0.05 m  d_out=0.1 m  L=1 m  th_cond_min=10 W/(K*m)  th_cond=8.9 W/(K*m)  th_cond_TLU=[413, 401, 392, 383, 371, 357, 342] W/(K*m)  temp_TLU=[200, 273, 400, 600, 800, 1000, 1200] K  T_specify=off  T_priority=None  T=0 K  T_nominal_specify=off  T_nominal_value=1  T_nominal_unit=K  Q_specify=off  Q_priority=None  Q=0 W  Q_nominal_specify=off  Q_nominal_value=1  Q_nominal_unit=W
  TIM18 : fl_lib/Thermal/Thermal Elements/Conductive Heat Transfer  thermal_type=foundation.enum.ConstantVariableTabulated.Constant  wall_geometry=foundation.enum.ConductionWallGeometry.Planar  area=0.1 m^2  thickness=0.001 in  d_in=0.05 m  d_out=0.1 m  L=1 m  th_cond_min=10 W/(K*m)  th_cond=9.4 W/(K*m)  th_cond_TLU=[413, 401, 392, 383, 371, 357, 342] W/(K*m)  temp_TLU=[200, 273, 400, 600, 800, 1000, 1200] K  T_specify=off  T_priority=None  T=0 K  T_nominal_specify=off  T_nominal_value=1  T_nominal_unit=K  Q_specify=off  Q_priority=None  Q=0 W  Q_nominal_specify=off  Q_nominal_value=1  Q_nominal_unit=W
  TIM19 : fl_lib/Thermal/Thermal Elements/Conductive Heat Transfer  thermal_type=foundation.enum.ConstantVariableTabulated.Constant  wall_geometry=foundation.enum.ConductionWallGeometry.Planar  area=0.1 m^2  thickness=0.001 in  d_in=0.05 m  d_out=0.1 m  L=1 m  th_cond_min=10 W/(K*m)  th_cond=8.9 W/(K*m)  th_cond_TLU=[413, 401, 392, 383, 371, 357, 342] W/(K*m)  temp_TLU=[200, 273, 400, 600, 800, 1000, 1200] K  T_specify=off  T_priority=None  T=0 K  T_nominal_specify=off  T_nominal_value=1  T_nominal_unit=K  Q_specify=off  Q_priority=None  Q=0 W  Q_nominal_specify=off  Q_nominal_value=1  Q_nominal_unit=W
  TIM20 : fl_lib/Thermal/Thermal Elements/Conductive Heat Transfer  thermal_type=foundation.enum.ConstantVariableTabulated.Constant  wall_geometry=foundation.enum.ConductionWallGeometry.Planar  area=0.1 m^2  thickness=0.001 in  d_in=0.05 m  d_out=0.1 m  L=1 m  th_cond_min=10 W/(K*m)  th_cond=8.9 W/(K*m)  th_cond_TLU=[413, 401, 392, 383, 371, 357, 342] W/(K*m)  temp_TLU=[200, 273, 400, 600, 800, 1000, 1200] K  T_specify=off  T_priority=None  T=0 K  T_nominal_specify=off  T_nominal_value=1  T_nominal_unit=K  Q_specify=off  Q_priority=None  Q=0 W  Q_nominal_specify=off  Q_nominal_value=1  Q_nominal_unit=W
  Thermal Reference{15..19} (5 alike) : fl_lib/Thermal/Thermal Elements/Thermal Reference
  Coolant In : PMIOPort  Side=Left
  Power In : PMIOPort  Port=2  Side=Left
  Coolant Out : PMIOPort  Port=3  Side=Right
  connections:
  TIM17/RConn1 -- Copper Thermal Mass13/LConn1 -- Copper Conduction 17/LConn1
  Copper Conduction 18/LConn1 -- TIM18/RConn1 -- Copper Thermal Mass14/LConn1
  Copper Conduction 20/LConn1 -- Copper Thermal Mass15/LConn1 -- TIM20/RConn1
  Copper Conduction 19/LConn1 -- Copper Thermal Mass3 3/LConn1 -- TIM19/RConn1
  Copper Conduction 16/LConn1 -- Copper Thermal Mass16/LConn1 -- TIM16/RConn1
  Thermal Reference16/LConn1 -- Controlled Heat Flow Rate Source16/RConn2
  Controlled Heat Flow Rate Source18/LConn1 -- IGBT20/LConn1
  Pipe (TL)3/LConn1 -- Pipe (TL)2/RConn1
  Pipe (TL)/LConn2 -- Copper Conduction 17/RConn1
  TIM19/LConn1 -- IGBT19/RConn1
  Controlled Heat Flow Rate Source15/LConn1 -- IGBT17/LConn1
  TIM20/LConn1 -- IGBT20/RConn1
  Controlled Heat Flow Rate Source17/LConn1 -- IGBT19/LConn1
  Controlled Heat Flow Rate Source16/LConn1 -- IGBT18/LConn1
  Pipe (TL)4/LConn1 -- Pipe (TL)3/RConn1
  Thermal Reference19/LConn1 -- Controlled Heat Flow Rate Source19/RConn2
  Pipe (TL)4/LConn2 -- Copper Conduction 16/RConn1
  TIM16/LConn1 -- IGBT16/RConn1
  Controlled Heat Flow Rate Source19/LConn1 -- IGBT16/LConn1
  Thermal Reference15/LConn1 -- Controlled Heat Flow Rate Source15/RConn2
  Pipe (TL)3/LConn2 -- Copper Conduction 20/RConn1
  Pipe (TL)2/LConn2 -- Copper Conduction 19/RConn1
  Thermal Reference17/LConn1 -- Controlled Heat Flow Rate Source17/RConn2
  Coolant In/RConn1 -- Pipe (TL)/LConn1
  Pipe (TL)1/LConn2 -- Copper Conduction 18/RConn1
  TIM17/LConn1 -- IGBT17/RConn1
  Pipe (TL)2/LConn1 -- Pipe (TL)1/RConn1
  TIM18/LConn1 -- IGBT18/RConn1
  Pipe (TL)1/LConn1 -- Pipe (TL)/RConn1
  Thermal Reference18/LConn1 -- Controlled Heat Flow Rate Source18/RConn2
  Pipe (TL)4/RConn1 -- Coolant Out/RConn1
  Power In/RConn1 -- Dividing it for 5 IGBT per Inverter/LConn1
  Dividing it for 5 IGBT per Inverter/RConn1 -- Controlled Heat Flow Rate Source15/RConn1 -- Controlled Heat Flow Rate Source16/RConn1 -- Controlled Heat Flow Rate Source19/RConn1 -- Controlled Heat Flow Rate Source18/RConn1 -- Controlled Heat Flow Rate Source17/RConn1
